simulink model "kbm_2020b"  (R2020b)
settings: Solver=VariableStepAuto  StartTime=0.0  StopTime=10.0  RelTol=1e-3
settings Model: Creator=felix  LastModifiedBy=Finn
settings DebuggingCC: SFMachineParentedDataDiag=error

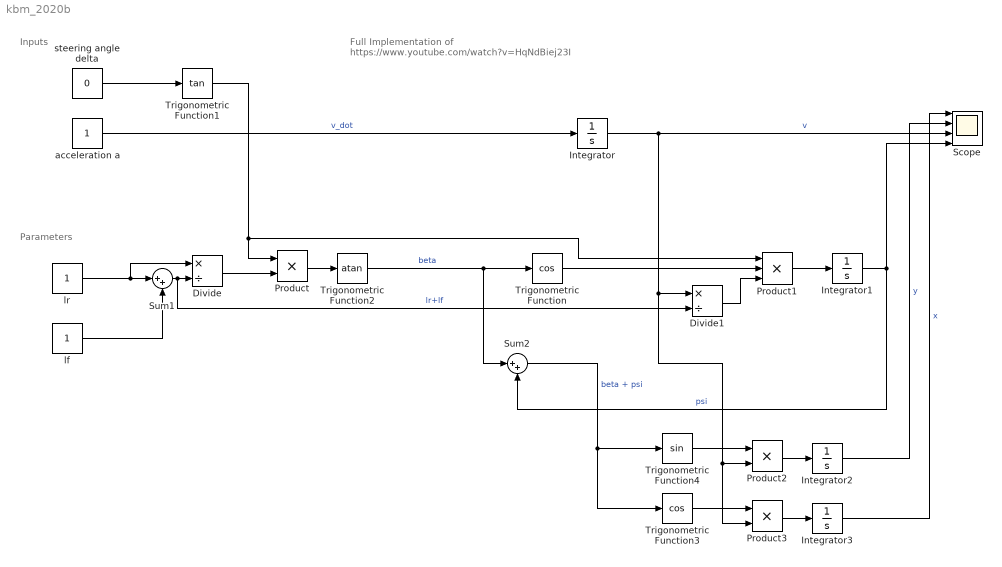
== system kbm_2020b ==
  note: Full Implementation of
      | https://www.youtube.com/watch?v=HqNdBiej23I
  note: Parameters
  note: Inputs
  Divide : Product  Inputs=*/
  Divide1 : Product  Inputs=*/
  Integrator{,1..3} (4 alike) : Integrator
  Product : Product
  Product1 : Product  Inputs=3
  Product2 : Product
  Product3 : Product
  Scope : Scope  NumInputPorts=4
  Sum1 : Sum  Inputs=|++
  Sum2 : Sum  Inputs=|++
  Trigonometric Function : Trigonometry  Operator=cos
  Trigonometric Function1 : Trigonometry  Operator=tan
  Trigonometric Function2 : Trigonometry  Operator=atan
  Trigonometric Function3 : Trigonometry  Operator=cos
  Trigonometric Function4 : Trigonometry
  acceleration a : Constant
  lf : Constant
  lr : Constant
  steering angle delta : Constant  Value=0
  wires:
  lr/1 -> Divide/1, Sum1/1
  lf/1 -> Sum1/2
  Sum1/1 -> Divide1/2, Divide/2  "lr+lf"
  Divide/1 -> Product/2
  steering angle delta/1 -> Trigonometric Function1/1
  Trigonometric Function1/1 -> Product1/1, Product/1
  Product/1 -> Trigonometric Function2/1
  acceleration a/1 -> Integrator/1  "v_dot"
  Integrator/1 -> Divide1/1, Product2/2, Product3/2, Scope/3  "v"
  Divide1/1 -> Product1/3
  Trigonometric Function2/1 -> Sum2/1, Trigonometric Function/1  "beta"
  Trigonometric Function/1 -> Product1/2
  Product1/1 -> Integrator1/1
  Integrator1/1 -> Scope/4, Sum2/2  "psi"
  Sum2/1 -> Trigonometric Function4/1, Trigonometric Function3/1  "beta + psi"
  Trigonometric Function4/1 -> Product2/1
  Trigonometric Function3/1 -> Product3/1
  Product2/1 -> Integrator2/1
  Product3/1 -> Integrator3/1
  Integrator3/1 -> Scope/1  "x"
  Integrator2/1 -> Scope/2  "y"
